simulink model "dk"  (R2022b)
settings: Solver=VariableStepAuto  StartTime=0.0  StopTime=1000  RelTol=1e-3
values from neighbouring files (symbols this model uses):
  A = J.A    [DK_iteration.m]    (also in Hinf_controller_Hinf.m = Jo.A; Hinf_controller_mixsyn.m = Jo.A; get_linearization.m = double(subs(A, [X(1);X(2);X(3);X(4);X(5);Tau(1);Tau(2)], [x_)
  B = J.B    [DK_iteration.m]    (also in Hinf_controller_Hinf.m = Jo.B; Hinf_controller_mixsyn.m = Jo.B; get_linearization.m = double(subs(B, [X(1);X(2);X(3);X(4);X(5);Tau(1);Tau(2)], [x_)
  C = J.C    [DK_iteration.m]    (also in Hinf_controller_Hinf.m = Jo.C; Hinf_controller_mixsyn.m = Jo.C; get_linearization.m = double(subs(C, [X(1);X(2);X(3);X(4);X(5);Tau(1);Tau(2)], [x_)
  D = J.D    [DK_iteration.m]    (also in Hinf_controller_Hinf.m = Jo.D; Hinf_controller_mixsyn.m = Jo.D; get_linearization.m = double(subs(D, [X(1);X(2);X(3);X(4);X(5);Tau(1);Tau(2)], [x_)
undefined symbols (not defined in the file or in its folder): A_DK, B_DK, C_DK, D_DK
settings Model: Creator=alexi  LastModifiedBy=alexi

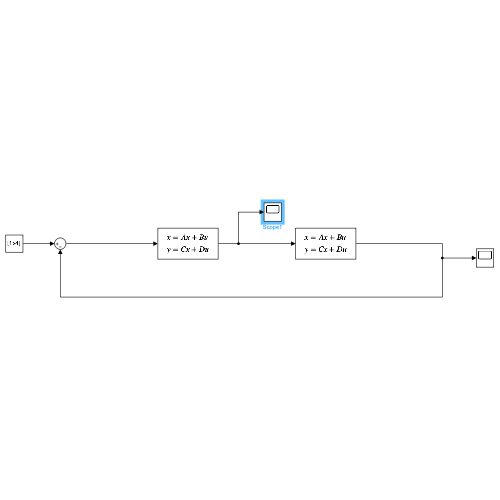
[thumbnail: Simulink's stored preview of the top-level diagram]
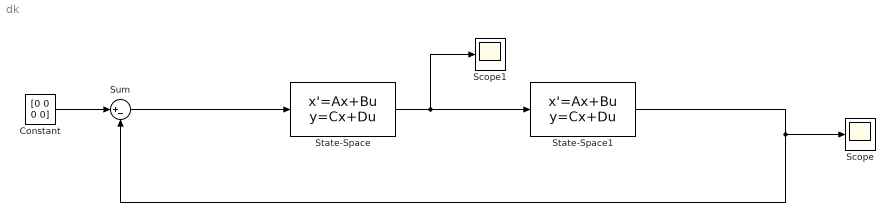
== system dk ==
  Constant : Constant  Value=[0 0 0 0]
  Scope : Scope
  Scope1 : Scope
  State-Space : StateSpace  A=A_DK  B=B_DK  C=C_DK  D=D_DK  InitialCondition=0
  State-Space1 : StateSpace  A=A  B=B  C=C  D=D  InitialCondition=[1 0 0 0 0]
  Sum : Sum  Inputs=|+-
  wires:
  State-Space/1 -> State-Space1/1, Scope1/1
  Constant/1 -> Sum/1
  Sum/1 -> State-Space/1
  State-Space1/1 -> Scope/1, Sum/2
